simulink model "Triangle_Connection_Capacitor_Compensation"  (Simulink 7.5)
settings: Solver=ode45  StartTime=0.0  StopTime=0.1  RelTol=1e-3
libraries: powerlib x22, powerlib_extras x1
settings Model: Creator=lm  LastModifiedBy=lm

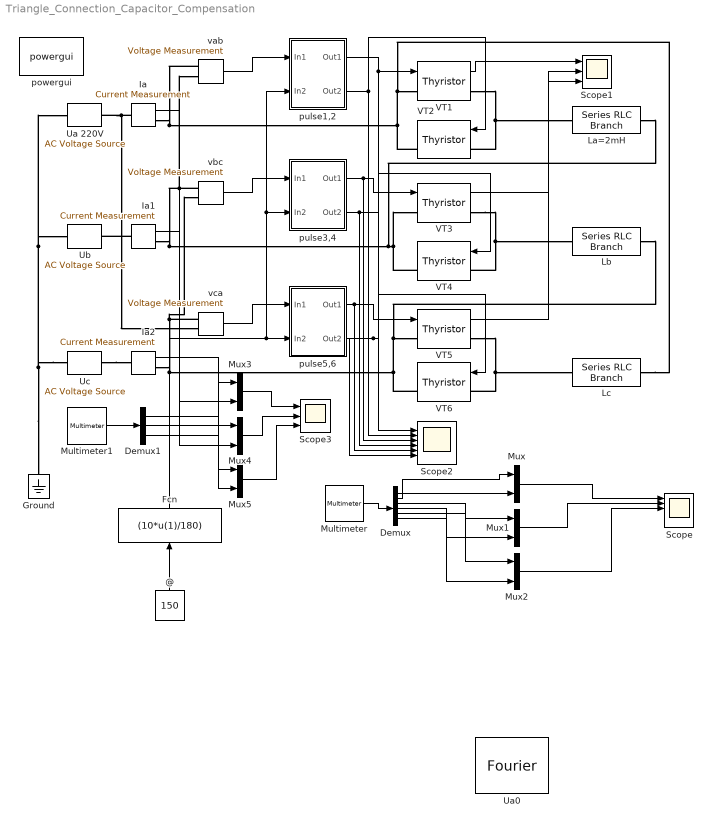
== system Triangle_Connection_Capacitor_Compensation ==
  @ : Constant  Value=150  OutDataType=fixdt(1, 16)  OutScaling=2^0
  Demux : Demux  Outputs=6
  Demux1 : Demux  Outputs=3
  Fcn : Fcn  Expr=(10*u(1)/180)
  Ground : powerlib/Elements/Ground  DialogController=POWERSYS.PowerSysDialog  PhysicalDomain=powersysdomain  SubClassName=unknown  LeftPortType=p1  RightPortType=p1  LConnTagsString=a
  Ia : powerlib/Measurements/Current Measurement  DialogController=POWERSYS.PowerSysDialog  SystemSampleTime=-1  PhasorSimulation=off  OutputType=Complex  PSBequivalent=0
  Ia1 : powerlib/Measurements/Current Measurement  DialogController=POWERSYS.PowerSysDialog  SystemSampleTime=-1  PhasorSimulation=off  OutputType=Complex  PSBequivalent=0
  Ia2 : powerlib/Measurements/Current Measurement  DialogController=POWERSYS.PowerSysDialog  SystemSampleTime=-1  PhasorSimulation=off  OutputType=Complex  PSBequivalent=0
  La=2mH : powerlib/Elements/Series RLC Branch  DialogController=POWERSYS.PowerSysDialog  PhysicalDomain=powersysdomain  SubClassName=unknown  LeftPortType=p1  RightPortType=p1  LConnTagsString=__new0  RConnTagsString=__new0  BranchType=L  Resistance=1  Inductance=2e-3  SetiL0=off  InitialCurrent=0  Capacitance=1e-6  Setx0=off  InitialVoltage=0  Measurements=Branch voltage and current
  Lb : powerlib/Elements/Series RLC Branch  DialogController=POWERSYS.PowerSysDialog  PhysicalDomain=powersysdomain  SubClassName=unknown  LeftPortType=p1  RightPortType=p1  LConnTagsString=__new0  RConnTagsString=__new0  BranchType=L  Resistance=1  Inductance=2e-3  SetiL0=off  InitialCurrent=0  Capacitance=1e-6  Setx0=off  InitialVoltage=0  Measurements=Branch voltage and current
  Lc : powerlib/Elements/Series RLC Branch  DialogController=POWERSYS.PowerSysDialog  PhysicalDomain=powersysdomain  SubClassName=unknown  LeftPortType=p1  RightPortType=p1  LConnTagsString=__new0  RConnTagsString=__new0  BranchType=L  Resistance=1  Inductance=2e-3  SetiL0=off  InitialCurrent=0  Capacitance=1e-6  Setx0=off  InitialVoltage=0  Measurements=Branch voltage and current
  Multimeter : powerlib/Measurements/Multimeter  SystemSampleTime=-1  PhasorSimulation=off  OutputType=Complex  sel=[1 7 2 8 3 9]  L=9  Gain=[1 1 1 1 1 1]  yselected={'Ub: La=2mH','Ib: La=2mH','Ub: Lb','Ib: Lb','Ub: Lc','Ib: Lc'};  PSBOutputType=1  PSBequivalent=0  AxesSetting=[0,0.1,-100,100]  Display=0  SavedBlockNames=-11
  Multimeter1 : powerlib/Measurements/Multimeter  SystemSampleTime=-1  PhasorSimulation=off  OutputType=Complex  sel=[6 5 4]  L=9  Gain=[1 1 1]  yselected={'Usrc: Ua 220V','Usrc: Ub','Usrc: Uc '};  PSBOutputType=1  PSBequivalent=0  AxesSetting=[0,0.1,-100,100]  Display=0  SavedBlockNames=-11
  Mux{,1..5} (6 alike) : Mux  Inputs=2
  Scope : Scope  NumInputPorts=6
      settings: YMin=-5~-5~-5~-5~-5~-5  YMax=5~5~5~5~5~5
  Scope1 : Scope  NumInputPorts=3
      settings: YMin=-5~-5~-5  YMax=5~5~5
  Scope2 : Scope  NumInputPorts=6
      settings: TimeRange=0.1  YMin=-0~0~0~0~0~0  YMax=2~2~2~2~2~2  SaveName=ScopeData2
  Scope3 : Scope  NumInputPorts=3
      settings: TimeRange=0.0002084291187739451  YMin=39.01041666666609~-2500~-400  YMax=199.0104166666661~500~1000  SaveName=ScopeData3
  Ua 220V : powerlib/Electrical Sources/AC Voltage Source  DialogController=POWERSYS.PowerSysDialog  SystemSampleTime=-1  Amplitude=220*sqrt(2)  Phase=0  Frequency=50  SampleTime=0  Measurements=Voltage
  Ua0 : powerlib_extras/Measurements/Fourier  DialogController=POWERSYS.PowerSysDialog  SystemSampleTime=-1  f1=50  n=0
  Ub : powerlib/Electrical Sources/AC Voltage Source  DialogController=POWERSYS.PowerSysDialog  SystemSampleTime=-1  Amplitude=220*sqrt(2)  Phase=-120  Frequency=50  SampleTime=0  Measurements=Voltage
  "Uc " : powerlib/Electrical Sources/AC Voltage Source  DialogController=POWERSYS.PowerSysDialog  SystemSampleTime=-1  Amplitude=220*sqrt(2)  Phase=-240  Frequency=50  SampleTime=0  Measurements=Voltage
  VT{1..6} (6 alike) : powerlib/Power Electronics/Thyristor  DialogController=POWERSYS.PowerSysDialog  SystemSampleTime=-1  Ron=0.001  Lon=0  Vf=0.8  IC=0  Rs=500  Cs=250e-9  Measurements=on
  powergui : powerlib/powergui  Priority=1  SystemSampleTime=-1  SimulationMode=Continuous  SampleTime=50e-6  frequency=60  SPID=off  DisableSnubberDevices=off  DisableRonSwitches=off  DisableVfSwitches=off  SwTol=0  Interpol=off  frequencyindice=50  echomessages=off  HookPort=off  DisplayEquations=off  FunctionMessages=off  EnableUseOfTLC=off  x0status=blocks  RestoreLinks=warning  ResistiveCurrentMeasurement=off  Ylog=off  Xlog=on  ShowGrid=off  save=off  variable=ZData  ZoomFFT=off  StartTime=0.0  cycles=1  DisplayStyle=1  FreqAxis=off  MaxFrequency=1000  frequencyindicesteady=1  display=off  methode=off
  pulse1,2 : Subsystem
  pulse3,4 : Subsystem
  pulse5,6 : Subsystem
  vab : powerlib/Measurements/Voltage Measurement  DialogController=POWERSYS.PowerSysDialog  SystemSampleTime=-1  PhasorSimulation=off  OutputType=Complex  PSBequivalent=0
  vbc : powerlib/Measurements/Voltage Measurement  DialogController=POWERSYS.PowerSysDialog  SystemSampleTime=-1  PhasorSimulation=off  OutputType=Complex  PSBequivalent=0
  vca : powerlib/Measurements/Voltage Measurement  DialogController=POWERSYS.PowerSysDialog  SystemSampleTime=-1  PhasorSimulation=off  OutputType=Complex  PSBequivalent=0
  wires:
  vab/1 -> pulse1,2/1(In1)
  vbc/1 -> pulse3,4/1(In1)
  vca/1 -> pulse5,6/1(In1)
  pulse1,2/1(Out1) -> VT1/1, Scope2/1
  pulse1,2/2(Out2) -> VT2/1, Scope2/2
  pulse3,4/1(Out1) -> VT3/1, Scope2/3
  pulse5,6/1(Out1) -> VT5/1, Scope2/5
  pulse3,4/2(Out2) -> VT4/1, Scope2/4
  pulse5,6/2(Out2) -> VT6/1, Scope2/6
  @/1 -> Fcn/1
  Fcn/1 -> pulse5,6/2(In2), pulse3,4/2(In2), pulse1,2/2(In2)
  Multimeter/1 -> Demux/1
  VT1/1 -> Scope1/1
  VT3/1 -> Scope1/2
  VT5/1 -> Scope1/3
  Demux/1 -> Mux/1
  Demux/2 -> Mux/2
  Demux/3 -> Mux1/1
  Demux/4 -> Mux1/2
  Demux/5 -> Mux2/1
  Demux/6 -> Mux2/2
  Mux/1 -> Scope/1
  Mux1/1 -> Scope/2
  Mux2/1 -> Scope/3
  Mux3/1 -> Scope3/1
  Mux4/1 -> Scope3/2
  Mux5/1 -> Scope3/3
  Ia/1 -> Mux3/2
  Ia1/1 -> Mux4/2
  Ia2/1 -> Mux5/2
  Multimeter1/1 -> Demux1/1
  Demux1/1 -> Mux3/1
  Demux1/2 -> Mux4/1
  Demux1/3 -> Mux5/1
  connections:
  VT2/RConn1 -- vab/LConn1 -- Ia/RConn1 -- VT1/LConn1 -- Lc/RConn1
  VT1/RConn1 -- VT2/LConn1 -- La=2mH/LConn1
  vbc/LConn1 -- Ia1/RConn1 -- VT4/RConn1 -- VT3/LConn1 -- La=2mH/RConn1 -- vab/LConn2
  VT3/RConn1 -- VT4/LConn1 -- Lb/LConn1
  VT5/RConn1 -- VT6/LConn1 -- Lc/LConn1
  vca/LConn1 -- VT6/RConn1 -- VT5/LConn1 -- Lb/RConn1 -- Ia2/RConn1 -- vbc/LConn2
  "Uc "/RConn1 -- Ia2/LConn1
  Ia1/LConn1 -- Ub/RConn1
  Ia/LConn1 -- Ua 220V/RConn1 -- vca/LConn2
  "Uc "/LConn1 -- Ua 220V/LConn1 -- Ub/LConn1 -- Ground/LConn1

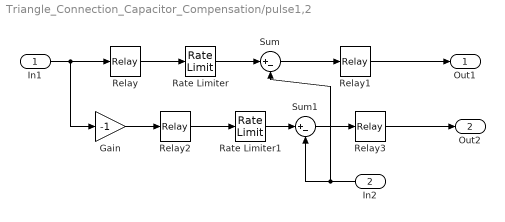
== system Triangle_Connection_Capacitor_Compensation/pulse1,2 ==
  In1 : Inport  OutDataType=fixdt(1, 16)  OutScaling=2^0
  In2 : Inport  Port=2  OutDataType=fixdt(1, 16)  OutScaling=2^0
  Gain : Gain  Gain=-1  ParameterDataType=fixdt(1, 16)  ParameterScaling=2^0  OutDataType=fixdt(1, 16)  OutScaling=2^0
  Rate Limiter : RateLimiter  RisingSlewLimit=1000  FallingSlewLimit=-1e8  SampleTimeMode=inherited
  Rate Limiter1 : RateLimiter  RisingSlewLimit=1000  FallingSlewLimit=-1e9  SampleTimeMode=inherited
  Relay : Relay  OnOutputValue=10  OutDataType=fixdt(1, 16)  OutScaling=2^0
  Relay1 : Relay  OutDataType=fixdt(1, 16)  OutScaling=2^0
  Relay2 : Relay  OnOutputValue=10  OutDataType=fixdt(1, 16)  OutScaling=2^0
  Relay3 : Relay  OutDataType=fixdt(1, 16)  OutScaling=2^0
  Sum : Sum  Inputs=|+-  OutDataType=fixdt(1, 16)  OutScaling=2^0
  Sum1 : Sum  Inputs=|+-  OutDataType=fixdt(1, 16)  OutScaling=2^0
  Out1 : Outport  OutDataType=fixdt(1, 16)  OutScaling=2^0
  Out2 : Outport  Port=2  OutDataType=fixdt(1, 16)  OutScaling=2^0
  wires:
  Rate Limiter/1 -> Sum/1
  Relay/1 -> Rate Limiter/1
  Relay3/1 -> Out2/1
  Sum1/1 -> Relay3/1
  In2/1 -> Sum/2, Sum1/2
  Rate Limiter1/1 -> Sum1/1
  Relay2/1 -> Rate Limiter1/1
  Gain/1 -> Relay2/1
  In1/1 -> Gain/1, Relay/1
  Sum/1 -> Relay1/1
  Relay1/1 -> Out1/1

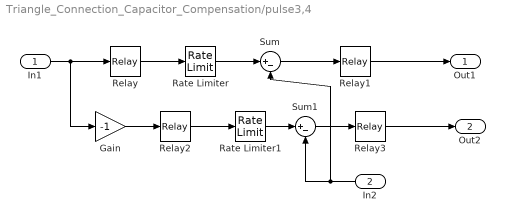
== system Triangle_Connection_Capacitor_Compensation/pulse3,4 ==
  In1 : Inport  OutDataType=fixdt(1, 16)  OutScaling=2^0
  In2 : Inport  Port=2  OutDataType=fixdt(1, 16)  OutScaling=2^0
  Gain : Gain  Gain=-1  ParameterDataType=fixdt(1, 16)  ParameterScaling=2^0  OutDataType=fixdt(1, 16)  OutScaling=2^0
  Rate Limiter : RateLimiter  RisingSlewLimit=1000  FallingSlewLimit=-1e8  SampleTimeMode=inherited
  Rate Limiter1 : RateLimiter  RisingSlewLimit=1000  FallingSlewLimit=-1e9  SampleTimeMode=inherited
  Relay : Relay  OnOutputValue=10  OutDataType=fixdt(1, 16)  OutScaling=2^0
  Relay1 : Relay  OutDataType=fixdt(1, 16)  OutScaling=2^0
  Relay2 : Relay  OnOutputValue=10  OutDataType=fixdt(1, 16)  OutScaling=2^0
  Relay3 : Relay  OutDataType=fixdt(1, 16)  OutScaling=2^0
  Sum : Sum  Inputs=|+-  OutDataType=fixdt(1, 16)  OutScaling=2^0
  Sum1 : Sum  Inputs=|+-  OutDataType=fixdt(1, 16)  OutScaling=2^0
  Out1 : Outport  OutDataType=fixdt(1, 16)  OutScaling=2^0
  Out2 : Outport  Port=2  OutDataType=fixdt(1, 16)  OutScaling=2^0
  wires:
  Relay1/1 -> Out1/1
  Sum/1 -> Relay1/1
  In1/1 -> Relay/1, Gain/1
  Gain/1 -> Relay2/1
  Relay2/1 -> Rate Limiter1/1
  Rate Limiter1/1 -> Sum1/1
  In2/1 -> Sum1/2, Sum/2
  Sum1/1 -> Relay3/1
  Relay3/1 -> Out2/1
  Relay/1 -> Rate Limiter/1
  Rate Limiter/1 -> Sum/1

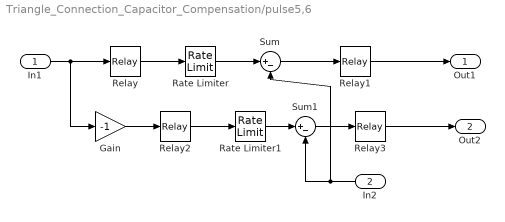
== system Triangle_Connection_Capacitor_Compensation/pulse5,6 ==
  In1 : Inport  OutDataType=fixdt(1, 16)  OutScaling=2^0
  In2 : Inport  Port=2  OutDataType=fixdt(1, 16)  OutScaling=2^0
  Gain : Gain  Gain=-1  ParameterDataType=fixdt(1, 16)  ParameterScaling=2^0  OutDataType=fixdt(1, 16)  OutScaling=2^0
  Rate Limiter : RateLimiter  RisingSlewLimit=1000  FallingSlewLimit=-1e8  SampleTimeMode=inherited
  Rate Limiter1 : RateLimiter  RisingSlewLimit=1000  FallingSlewLimit=-1e9  SampleTimeMode=inherited
  Relay : Relay  OnOutputValue=10  OutDataType=fixdt(1, 16)  OutScaling=2^0
  Relay1 : Relay  OutDataType=fixdt(1, 16)  OutScaling=2^0
  Relay2 : Relay  OnOutputValue=10  OutDataType=fixdt(1, 16)  OutScaling=2^0
  Relay3 : Relay  OutDataType=fixdt(1, 16)  OutScaling=2^0
  Sum : Sum  Inputs=|+-  OutDataType=fixdt(1, 16)  OutScaling=2^0
  Sum1 : Sum  Inputs=|+-  OutDataType=fixdt(1, 16)  OutScaling=2^0
  Out1 : Outport  OutDataType=fixdt(1, 16)  OutScaling=2^0
  Out2 : Outport  Port=2  OutDataType=fixdt(1, 16)  OutScaling=2^0
  wires:
  Rate Limiter/1 -> Sum/1
  Relay/1 -> Rate Limiter/1
  Relay3/1 -> Out2/1
  Sum1/1 -> Relay3/1
  In2/1 -> Sum/2, Sum1/2
  Rate Limiter1/1 -> Sum1/1
  Relay2/1 -> Rate Limiter1/1
  Gain/1 -> Relay2/1
  In1/1 -> Gain/1, Relay/1
  Sum/1 -> Relay1/1
  Relay1/1 -> Out1/1
